simulink model "MBSE_Project_SeatBeltRemainder_Manual"  (R2020b)
settings: Solver=VariableStepAuto  StartTime=0.0  StopTime=inf  RelTol=1e-3
settings Model: Creator=99003747  LastModifiedBy=99003747

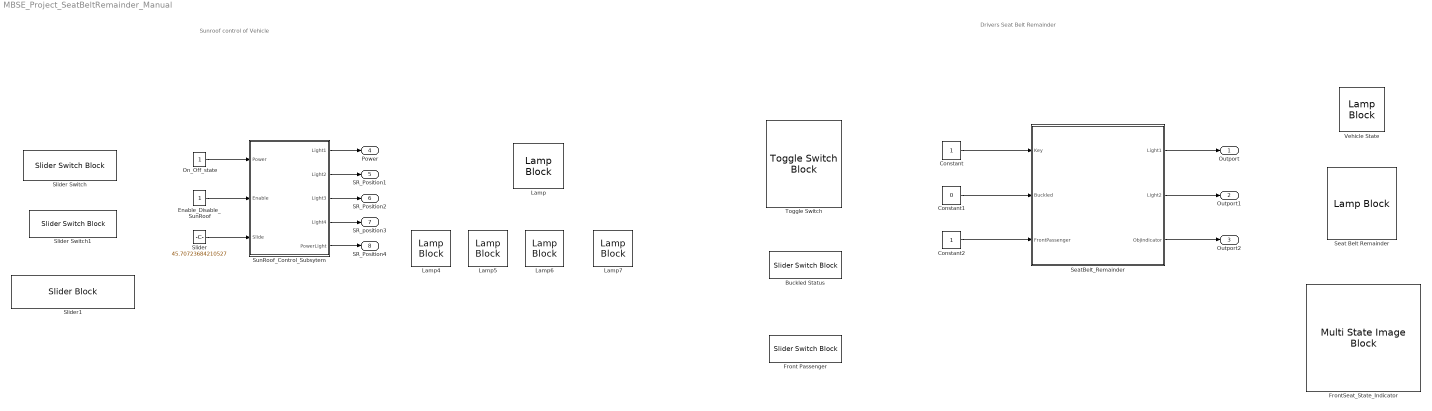
== system MBSE_Project_SeatBeltRemainder_Manual ==
  note: Drivers Seat Belt Remainder
  note: Sunroof control of Vehicle
  Buckled Status : SliderSwitchBlock
      settings: Values={{'Off', 'On'}, [0 1]}
  Constant : Constant
  Constant1 : Constant  Value=0
  Constant2 : Constant
  Enable_Disable_SunRoof : Constant
  Front Passenger : SliderSwitchBlock
      settings: Values={{'Off', 'On'}, [0 1]}
  FrontSeat_State_Indicator : MultiStateImageBlock
  Lamp{,4..7} (5 alike) : LampBlock
  On_Off_state : Constant
  Seat Belt Remainder : LampBlock
  SeatBelt_Remainder : Stateflow chart  TreatAsAtomicUnit=on
  Slider : Constant  Value=45.70723684210527
  Slider Switch : SliderSwitchBlock
      settings: Values={{'Off', 'On'}, [0 1]}
  Slider Switch1 : SliderSwitchBlock
      settings: Values={{'Off', 'On'}, [0 1]}
  Slider1 : SliderBlock
  SunRoof_Control_Subsytem : Subsystem
      mask Display: image('C:\Users\99003747\Desktop\sunroof.jfif')
  Toggle Switch : ToggleSwitchBlock
      settings: Values={{'Off', 'On'}, [0 1]}
  Vehicle State : LampBlock
  Outport : Outport
  Outport1 : Outport  Port=2
  Outport2 : Outport  Port=3
  Power : Outport  Port=4
  SR_Position1 : Outport  Port=5
  SR_Position2 : Outport  Port=6
  SR_position3 : Outport  Port=7
  SR_Position4 : Outport  Port=8
  wires:
  SeatBelt_Remainder/1(Light1) -> Outport/1
  SeatBelt_Remainder/2(Light2) -> Outport1/1
  Constant/1 -> SeatBelt_Remainder/1(Key)
  Constant1/1 -> SeatBelt_Remainder/2(Buckled)
  Constant2/1 -> SeatBelt_Remainder/3(FrontPassenger)
  SeatBelt_Remainder/3(ObjIndicator) -> Outport2/1
  SunRoof_Control_Subsytem/5(PowerLight) -> SR_Position4/1
  SunRoof_Control_Subsytem/2(Light2) -> SR_Position1/1
  Slider/1 -> SunRoof_Control_Subsytem/3(Slide)
  SunRoof_Control_Subsytem/3(Light3) -> SR_Position2/1
  SunRoof_Control_Subsytem/4(Light4) -> SR_position3/1
  On_Off_state/1 -> SunRoof_Control_Subsytem/1(Power)
  SunRoof_Control_Subsytem/1(Light1) -> Power/1
  Enable_Disable_SunRoof/1 -> SunRoof_Control_Subsytem/2(Enable)

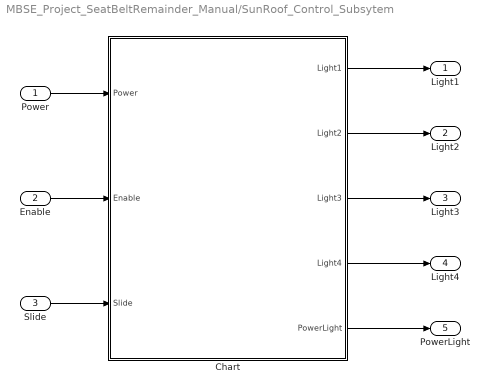
== system MBSE_Project_SeatBeltRemainder_Manual/SunRoof_Control_Subsytem ==
  Power : Inport
  Enable : Inport  Port=2
  Slide : Inport  Port=3
  Chart : Stateflow chart  TreatAsAtomicUnit=on
  Light1 : Outport
  Light2 : Outport  Port=2
  Light3 : Outport  Port=3
  Light4 : Outport  Port=4
  PowerLight : Outport  Port=5
  wires:
  Slide/1 -> Chart/3(Slide)
  Chart/3(Light3) -> Light3/1
  Chart/1(Light1) -> Light1/1
  Chart/2(Light2) -> Light2/1
  Enable/1 -> Chart/2(Enable)
  Power/1 -> Chart/1(Power)
  Chart/4(Light4) -> Light4/1
  Chart/5(PowerLight) -> PowerLight/1

== stateflow chart MBSE_Project_SeatBeltRemainder_Manual/SunRoof_Control_Subsytem/Chart ==
  state PowerOff
    entry:
    PowerLight=0;
    Light1=0;
    Light2=0;
    Light3=0;
    Light4=0;
  state PowerOn
    entry:
    PowerLight=1;
    Light1=0;
    Light2=0;
    Light3=0;
    Light4=0;
  state RoofPosition1
    entry:
    Light1=1;
    Light2=0;
    Light3=0;
    Light4=0;
  state RoofPosition2
    entry:
    Light1=1;
    Light2=1;
    Light3=0;
    Light4=0;
  state RoofPosition4
    entry:
    Light1=1;
    Light2=1;
    Light3=1;
    Light4=1;
  state RoofPosition3
    entry:
    Light1=1;
    Light2=1;
    Light3=1;
    Light4=0;
  (default) -> PowerOff
  PowerOn -> RoofPosition4 [order 2] : [Enable ==1 && Slide>75 && Slide<=100]
  PowerOff -> PowerOn : [Power == 1  ]
  RoofPosition4 -> PowerOn [order 1] : [Enable == 0]
  PowerOn -> PowerOff [order 5] : [Power == 0]
  RoofPosition1 -> PowerOn [order 4] : [Enable ==1 && Slide<=0 && Slide>25]
  PowerOn -> RoofPosition1 [order 4] : [Enable ==1 && Slide>0 && Slide<25]
  RoofPosition1 -> PowerOff [order 2] : [Power == 0]
  RoofPosition1 -> PowerOn [order 1] : [Enable == 0]
  RoofPosition4 -> PowerOff [order 2] : [Power == 0]
  PowerOn -> RoofPosition2 [order 3] : [Enable ==1 && Slide>=25 && Slide<50]
  RoofPosition2 -> PowerOn [order 1] : [Enable == 0]
  RoofPosition3 -> PowerOn [order 1] : [Enable == 0]
  PowerOn -> RoofPosition3 [order 1] : [Enable ==1 && Slide>=50 && Slide<75]
  RoofPosition2 -> PowerOff [order 2] : [Power == 0]
  RoofPosition3 -> PowerOff [order 2] : [Power == 0]
  RoofPosition2 -> RoofPosition1 [order 3] : [Enable ==1 && Slide<=25 && Slide>0]
  RoofPosition3 -> RoofPosition2 [order 3] : [Enable ==1 && Slide<=50 && Slide>25]
  RoofPosition4 -> RoofPosition3 [order 3] : [Enable ==1 && Slide<=75 && Slide>50]
  RoofPosition1 -> RoofPosition2 [order 3] : [Enable ==1 && Slide>=25 && Slide<50]
  RoofPosition2 -> RoofPosition3 [order 4] : [Enable ==1 && Slide>=50 && Slide<75]
  RoofPosition3 -> RoofPosition4 [order 4] : [Enable ==1 && Slide>=75 && Slide<100]
  data: Power input; Light1 output; Enable input; Light2 output; Light3 output; Light4 output; Slide input; PowerLight output

== stateflow chart MBSE_Project_SeatBeltRemainder_Manual/SeatBelt_Remainder ==
  state Indicator
    entry:
    ObjIndicator=1;
    state VehicleOn
      entry:
      Light1=1;
      Light2=1;
    state Chime
      entry:
      Light2=0;
    (default) -> VehicleOn
    Chime -> VehicleOn : [Light2==0]
    VehicleOn -> Chime : [Light2==1]
  state VehicleOff
    entry:
    Light1=0;
    Light2=0;
  state SeatBeltBuckled
    entry:
    Light2=0;
  state frontPassenger
    entry:
    ObjIndicator=0;
  (default) -> VehicleOff
  Indicator -> SeatBeltBuckled [order 1] : [Buckled==1]
  Indicator -> VehicleOff [order 3] : [Key==0]
  SeatBeltBuckled -> Indicator [order 1] : [Buckled==0]
  VehicleOff -> Indicator : [Key==1 ]
  SeatBeltBuckled -> VehicleOff [order 2] : [Key==0]
  frontPassenger -> SeatBeltBuckled [order 2] : [Buckled == 1]
  SeatBeltBuckled -> frontPassenger [order 3] : [Buckled == 0]
  frontPassenger -> Indicator [order 1] : [Key == 1 && FrontPassenger ==1 ]
  Indicator -> frontPassenger [order 2] : [ FrontPassenger ==0]
  frontPassenger -> VehicleOff [order 3] : [Key == 0]
  data: Light1 output; Light2 output; Key input =0; Buckled input; ObjIndicator output; FrontPassenger input
